simulink model "led_blink_sl_analog"  (R2022b)
settings: Solver=VariableStepAuto  StartTime=0.0  StopTime=10.0  RelTol=1e-3
libraries: arduino_io_lib x3
settings Model: Creator=user  LastModifiedBy=user

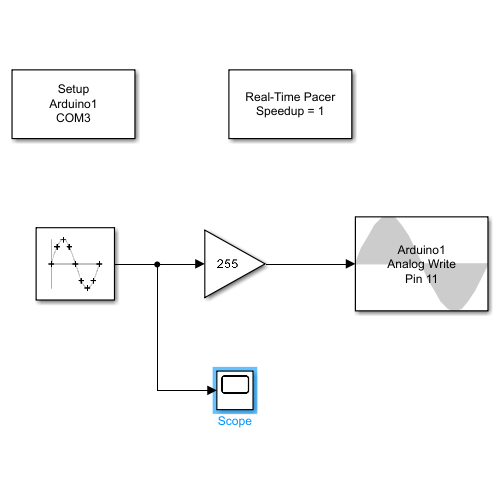
[thumbnail: Simulink's stored preview of the top-level diagram]
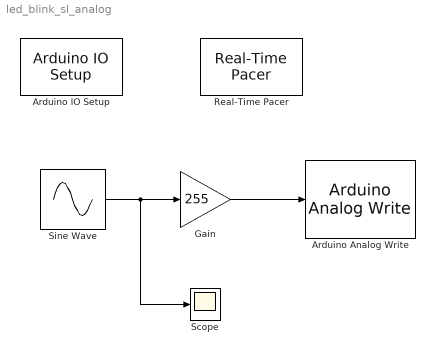
== system led_blink_sl_analog ==
  Arduino Analog Write : arduino_io_lib/Arduino Analog Write  arduinoVar=Temporary arduino variable: Arduino1  arduinoPin=11  T=0.2
  Arduino IO Setup : arduino_io_lib/Arduino IO Setup  Priority=3  arduinoVar=Temporary arduino variable: Arduino1  workspaceVarName=a  comPort=COM3
  Gain : Gain  Gain=255
  Real-Time Pacer : arduino_io_lib/Real-Time Pacer  simTimePerRealTime=1
  Scope : Scope
  Sine Wave : Sin  SineType=Sample based  Amplitude=0.5  Bias=0.5  Samples=50  SampleTime=0.02
  wires:
  Gain/1 -> Arduino Analog Write/1
  Sine Wave/1 -> Scope/1, Gain/1
